simulink model "Mux3"  (R2023b)
settings: Solver=VariableStepAuto  StartTime=0.0  StopTime=10.0  RelTol=1e-3
settings Model: Creator=DarianMuresan  LastModifiedBy=iceki

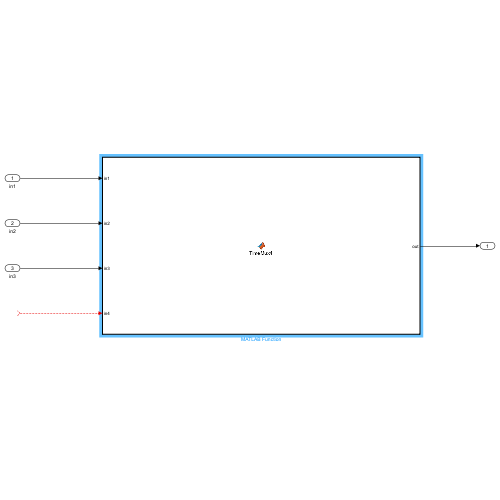
[thumbnail: Simulink's stored preview of the top-level diagram]
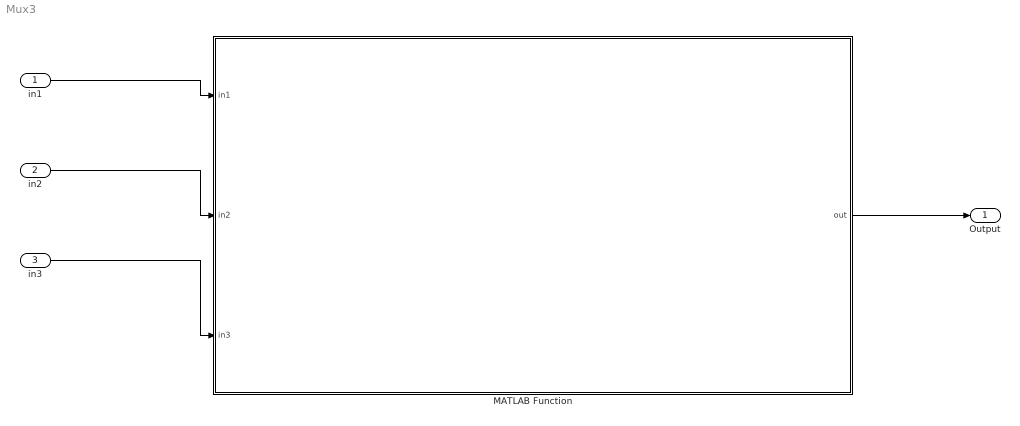
== system Mux3 ==
  in1 : Inport
  in2 : Inport  Port=2
  in3 : Inport  Port=3
  MATLAB Function : MATLAB Function  TreatAsAtomicUnit=on
  Output : Outport
  wires:
  ? -> ?
  in3/1 -> MATLAB Function/3(in3)
  in2/1 -> MATLAB Function/2(in2)
  in1/1 -> MATLAB Function/1(in1)
  MATLAB Function/1(out) -> Output/1

== matlab function Mux3/MATLAB Function ==
  data: in1 input; out output; in2 input; in3 input
function out = TimeMux4(in1,in2,in3)

% Method to mux 3 inputs into one of 3 possible outputs based on
% the first non-negative input.
%
% Written by: Darian Muresan
% Last Modified: 10/17/2023

if nargin<2
    in2=-1;
    in3=-1;
elseif nargin<3
    in3=-1;
end

if in1>=0
    out = in1;
elseif in2>=0
    out = in2;
elseif in3>=0
    out = in3;
else
    out = -1;
end
